simulink model "NDO_STO_KDO_2_2017b"  (R2017b)
settings: Solver=FixedStepAuto  StartTime=0.0  StopTime=100  FixedStep=0.001  RelTol=1e-3
undefined symbols (not defined in the file or in its folder): B, k1, k2, k3, k4, k5, k6, MI
libraries: powerlib_extras x21, commchan3 x15, simulink x4, checkpacklib x2
(part 3 of 3)

== matlab function NDO_STO_KDO_2_2017b/ Kernel Differentiator Observer/MATLAB Function ==
  data: x input; x_window output; x_prev input; t input
function x_window  = fcn(x, x_prev, t)
x_window = [x_prev(2:end,:); x(1) x(3) x(5) x(7) x(9) x(11) t];

== matlab function NDO_STO_KDO_2_2017b/ Kernel Differentiator Observer/ 1 ==
  data: U1 input; U2 input; U3 input; U4 input; uxa input; uya input; w input; x input; xp input; x_estimate input; xp_estimate input; params input; dis_z_est output; dis_x_est output; dis_y_est output; dis_fi_est output; dis_th_est output; dis_ya_est output; params output
function [dis_z_est,dis_x_est,dis_y_est,dis_fi_est,dis_th_est,dis_ya_est, params]= fcn(U1,U2,U3,U4,uxa,uya,w,x,xp, x_estimate, xp_estimate, params)

%%******************** parametrs *************
m=0.0296;
Ix=2.098*10^-5;
Iy=2.12*10^-5;
Iz=3.269*10^-5;
d=0.3;
g=9.81;
JR=(0.5*0.0025*23.1348*10^-3*23.1348*10^-3);
b=2.98*10^-5;
c=1.140*10^-7;
l=39.73*10^-3;

a1=(Iy-Iz)/Ix;
a2=-JR/Ix;
a3=(Iz-Ix)/Iy;
a4=JR/Iy;
a5=(Ix-Iy)/Iz;
b1=1/Ix;
b2=1/Iy;
b3=1/Iz;

% % If array has not been completely collected then output disturbances as
% % zero
% if x(end, 7)<25 % x(1,7)==0 &&
%     dis_z_est = 0;
%     dis_x_est = 0;
%     dis_y_est = 0; 
%     dis_fi_est = 0;
%     dis_th_est = 0;
%     dis_ya_est = 0;
%     return
% end
% 
% 
% 
% % Read the states from window
% phi_array = x(:,1); theta_array = x(:,2); psi_array = x(:,3);
% z_array = x(:,4); x_array = x(:,5); y_array = x(:,6); t_array = x(:,7);
% phi_param = params(:,1); theta_param =params(:,2); psi_param = params(:,3);
% z_param = params(:,4); x_param = params(:,5); y_param = params(:,6);
% 
% u = zeros(1,51); max_count=1000;
% %options = optimoptions('fminunc', 'MaxIterations', 20, 'UseParallel' ,true);
% 
% % Return if the latest time instant isnt a multiple of 0.025
% % This is there to reduce the number of computations
% if mod(x(end, 7), 0.025)==0
%     % Phi Estimation
%     ff = @(w)cost_func_sync_gen(w, phi_param, t_array, phi_array, u);
%     phi_param = fminsearch(ff, phi_param);
%     % theta Estimation
%     ff = @(w)cost_func_sync_gen(w, theta_param, t_array, theta_array, u);
%     theta_param = fminsearch(ff, theta_param);
%     % Psi Estimation
%     ff = @(w)cost_func_sync_gen(w, psi_param, t_array, psi_array, u);
%     psi_param = fminsearch(ff, psi_param);
%     % Z Estimation
%     ff = @(w)cost_func_sync_gen(w, z_param, t_array, z_array, u);
%     z_param = fminsearch(ff, z_param);
%     % X Estimation
%     ff = @(w)cost_func_sync_gen(w, x_param, t_array, x_array, u);
%     x_param = fminsearch(ff, x_param);
%     % Y Estimation
%     ff = @(w)cost_func_sync_gen(w, y_param, t_array, y_array, u);
%     y_param = fminsearch(ff, z_param);
% end
% 
% [phi_est_win, phi_dot_est_win, phi_ddot_est_win, ~] = output_point_estimator(t_array(end), phi_array, u, t_array(1), t_array(end), phi_param, max_count);
% [theta_est_win, theta_dot_est_win, theta_ddot_est_win, ~] = output_point_estimator(t_array(end), theta_array, u, t_array(1), t_array(end), theta_param, max_count);
% [psi_est_win, psi_dot_est_win, psi_ddot_est_win, ~] = output_point_estimator(t_array(end), psi_array, u, t_array(1), t_array(end), psi_param, max_count);
% [~, ~, z_ddot_est_win, ~] = output_point_estimator(t_array(end), z_array, u, t_array(1), t_array(end), z_param, max_count);
% [~, ~, x_ddot_est_win, ~] = output_point_estimator(t_array(end), x_array, u, t_array(1), t_array(end), x_param, max_count);
% [~, ~, y_ddot_est_win, ~] = output_point_estimator(t_array(end), y_array, u, t_array(1), t_array(end), y_param, max_count);
% 
% params = [phi_param theta_param psi_param z_param x_param y_param];
% 
% phi=phi_est_win(end); phi_dot= phi_dot_est_win(end); phi_ddot=phi_ddot_est_win(end);
% theta=theta_est_win(end); theta_dot=theta_dot_est_win(end); theta_ddot=theta_ddot_est_win(end);
% psi = psi_est_win(end); psi_dot=psi_dot_est_win(end); psi_ddot=psi_ddot_est_win(end);
% z_ddot=z_ddot_est_win(end);
% x_ddot=x_ddot_est_win(end);
% y_ddot=y_ddot_est_win(end);


% param = param^3;
xp_estimate=xp(1:12); x_estimate = x; phi=x_estimate(1); 
phi_dot= x_estimate(2); phi_ddot=xp_estimate(2);
theta=x_estimate(3); theta_dot=x_estimate(4); theta_ddot=xp_estimate(4);
psi_dot=x_estimate(6); psi_ddot=xp_estimate(6);
z_ddot=xp_estimate(8);
x_ddot=xp_estimate(10);
y_ddot=xp_estimate(12);

% ux=cos(phi)*sin(theta)*cos(psi)+sin(phi)*sin(psi);
% uy=cos(phi)*sin(theta)*sin(psi)-sin(phi)*cos(psi);

dis_z_est = z_ddot - (-g+cos(phi)*cos(theta)*(1/m)*U1);
dis_x_est = x_ddot - ((uxa/m)*U1);
dis_y_est = y_ddot - ((uya/m)*U1);

dis_fi_est = phi_ddot - (theta_dot*psi_dot*a1 + theta_dot*a2*w + b1*U2);
dis_th_est = theta_ddot - (phi_dot*psi_dot*a3 + phi_dot*a4*w + b2*U3);
dis_ya_est = psi_ddot - (theta_dot*phi_dot*a5 + b3*U4);

% dis_z_est = 0;
% dis_x_est = 0;
% dis_y_est = 0; 
% dis_fi_est = 0;
% dis_th_est = 0;
% dis_ya_est = 0;
